simulink model "TrailerSoftware"  (R2019b)
settings: Solver=FixedStepDiscrete  StartTime=0.0  StopTime=inf  FixedStep=update  RelTol=1e-3  EnableMultiTasking=on
values from neighbouring files (symbols this model uses):
  countmax1 = 2500    [ProductionMfile.m]
  countmax2 = 2500    [ProductionMfile.m]
  HeaterIntGain = .0008    (= 0.0008)    [ProductionMfile.m]
  HeatGain = 10    [ProductionMfile.m]
  Intll = 0    [ProductionMfile.m]
  MaxCondPressure = 350    [ProductionMfile.m]
  MinSP = 1    [ProductionMfile.m]
  PostGain100 = 0.0002    [ProductionMfile.m]
  PostGain150 = 0.0005    [ProductionMfile.m]
  PostGain200 = 0.0004    [ProductionMfile.m]
  PostGain300 = 0.0008    [ProductionMfile.m]
  PostInit150 = 12    [ProductionMfile.m]
  PostIntulC = 65    [ProductionMfile.m]
  PostPGain = 0    [ProductionMfile.m]
  PreGain100 = 0.0005    [ProductionMfile.m]
  PreGain150 = 0.0005    [ProductionMfile.m]
  PreGain200 = 0.0003    [ProductionMfile.m]
  PreGain300 = 0.0008    [ProductionMfile.m]
  PreInit150 = 30    [ProductionMfile.m]
  PreIntulC = 65    [ProductionMfile.m]
  PreIntulDH = 65    [ProductionMfile.m]
  PrePGain = 0    [ProductionMfile.m]
  SatPress = [10 20 30 40 50 60 70 80 90 100 110 120 130 140 150 160 170      180 190 200 210 220 230 240 250 260 270 280 290 300 310 320 330      340 350 360 370 380 390 400 410 420 430 440 450 460 470 480 490      500]    [ProductionMfile.m]
  SatTemp = [-29.497 -2.4046 15.401 29.047 40.267 49.88 58.338 65.922 72.819      79.159 85.037 90.526 95.68 100.55 105.16 109.54 113.73 117.73 121.57      125.26 128.82 132.25 135.56 138.77 141.88 144.89 147.82 150.67 153.44      156.15 158.78 161.35 163.85 166.3 168.7 171.04 173.33 175.58 177.77      179.93 182.04 184.11 186.14 188.14 190.09 192.01 193.9 195.75 197.58      199.37]    [ProductionMfile.m]
  SHGain = 2    [ProductionMfile.m]
  SizeCANMatrix = 80    [ProductionMfile.m]
  SizeCOBIDVector = 10    [ProductionMfile.m]
  update = 0.002    [ProductionMfile.m]
undefined symbols (not defined in the file or in its folder): DiscIntNeverNeededParam, PostDGain, PreDGain, Ratio100, Ratio150, Ratio200, Ratio300
libraries: simulink x60, c2837xDlib x35, xpcutilitieslib x24, c2802xlib x8, c280xlib x7, etargetslib x4, svdutilitieslib x2, c2000lib x1
(part 2 of 8)

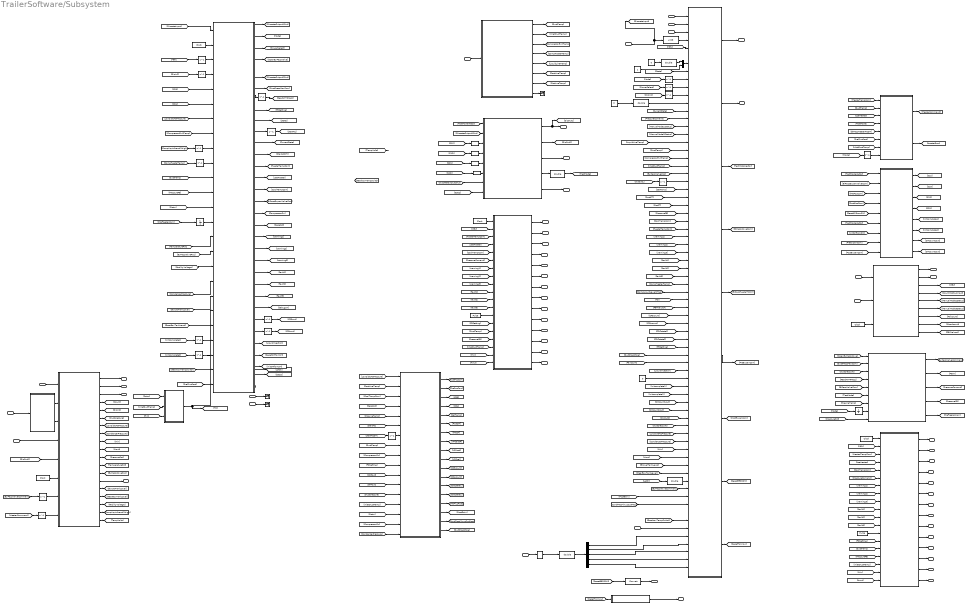
== system TrailerSoftware/Subsystem ==
  UDP Input Vector : Inport  OutDataTypeStr=uint8  PortDimensions=SizeUDPInput  SampleTime=update  LockScale=on
  A/D Vector : Inport  Port=2  PortDimensions=ADInputSize  SampleTime=update
  Discrete Input Word : Inport  Port=3  OutDataTypeStr=boolean  PortDimensions=DiscreteInputSize  SampleTime=update
  Modbus Input Vector : Inport  Port=4  OutDataTypeStr=uint8  PortDimensions=ModbusInputSize  SampleTime=update
  Modbus Input Ready : Inport  Port=5  OutDataTypeStr=uint8  PortDimensions=1  SampleTime=update
  UDP Input Ready : Inport  Port=6  OutDataTypeStr=boolean  PortDimensions=1  SampleTime=update
  CPUUtilizationsec : Inport  Port=7  OutDataTypeStr=double  PortDimensions=1  SampleTime=update
  EEPROM Input Vector : Inport  Port=8  OutDataTypeStr=single  PortDimensions=EEPROMSize  SampleTime=update
  New CAN Message : Inport  Port=9  OutDataTypeStr=uint8  SampleTime=update
  CAN Message Matrix : Inport  Port=10  OutDataTypeStr=uint8  PortDimensions=[1 SizeCANMatrix]  SampleTime=update
  CAN COBID Vector : Inport  Port=11  OutDataTypeStr=uint32  PortDimensions=[1 SizeCOBIDVector]  SampleTime=update
  RTD1 : Inport  Port=12  OutDataTypeStr=uint16  PortDimensions=1  SampleTime=update
  RTD2 : Inport  Port=13  OutDataTypeStr=uint16  PortDimensions=1  SampleTime=update
  WatchDogReset : Inport  Port=14  OutDataTypeStr=uint8  PortDimensions=1  SampleTime=update
  RomTestFailed : Inport  Port=15  OutDataTypeStr=uint8  PortDimensions=1  SampleTime=update
  CAN Process : MATLAB Function  TreatAsAtomicUnit=on
  Constant1 : Constant
  Constant2 : Constant  Value=0
  Constant4 : Constant  Value=0
  Constant9 : Constant  Value=0
  Data Type Conversion{1,8,10,12..13} (5 alike) : DataTypeConversion
  Data Type Conversion{2..3,6..7,9} (5 alike) : DataTypeConversion  OutDataTypeStr=double
  Data Type Conversion4 : DataTypeConversion  OutDataTypeStr=uint8
  Delay{,1..8,11..19} (18 alike) : Delay  DelayLength=1  InitialCondition=0
  Demux : Demux  Outputs=5
  Dew Point Temp : MATLAB Function  TreatAsAtomicUnit=on
  Digital Clock{,1..4} (5 alike) : DigitalClock  SampleTime=update
  Display : MATLAB Function  TreatAsAtomicUnit=on
  Display1 : MATLAB Function  TreatAsAtomicUnit=on
  Duct Pressure Control : Subsystem
  Heating : Subsystem
  MATLAB Function : MATLAB Function  TreatAsAtomicUnit=on
  Modbus Routine : MATLAB Function  TreatAsAtomicUnit=on
  Mux : Mux  Inputs=2
  Output Discrete : Subsystem
  Pulse Generator1 : DiscretePulseGenerator  Period=250  SampleTime=update
  Pulse Generator2 : DiscretePulseGenerator  Period=250  SampleTime=update
  Selector : Selector  InputPortWidth=32  IndexOptions=Index vector (dialog)  Indices=[28 29 30 31 32 ]  OutputSizes=1
  State Machine : MATLAB Function  TreatAsAtomicUnit=on
  Stepper Motor Reoutine : Subsystem
  Super Heat Control : Subsystem
  Temperature Vector : Subsystem
  Terminator3 : Terminator
  Terminator5 : Terminator
  Terminator6 : Terminator
  UDP Processing : Subsystem
  Unit Delay1 : UnitDelay  SampleTime=-1  HasFrameUpgradeWarning=on
  Unit Delay2 : UnitDelay  SampleTime=-1  HasFrameUpgradeWarning=on
  Unpack Data : Subsystem
  UDP Output Vector : Outport  OutDataTypeStr=uint8  PortDimensions=SizeUDPOutput  VectorParamsAs1DForOutWhenUnconnected=off  LockScale=on
  "Discrete Output Vector " : Outport  Port=2  OutDataTypeStr=uint8  PortDimensions=DiscreteOutputSize  SampleTime=update  VectorParamsAs1DForOutWhenUnconnected=off
  Modbus Output Vector : Outport  Port=3  OutDataTypeStr=uint8  PortDimensions=SizeModbusOutput  VectorParamsAs1DForOutWhenUnconnected=off  LockScale=on
  "HC Discrete Output Vector " : Outport  Port=4  OutDataTypeStr=uint8  PortDimensions=HCDiscreteOutputSize  SampleTime=update  VectorParamsAs1DForOutWhenUnconnected=off  LockScale=on
  Modbus Output Ready : Outport  Port=5  OutDataTypeStr=uint8  PortDimensions=1  SampleTime=update  VectorParamsAs1DForOutWhenUnconnected=off  LockScale=on
  UDP Output Ready : Outport  Port=6  OutDataTypeStr=uint8  SampleTime=update  VectorParamsAs1DForOutWhenUnconnected=off  LockScale=on
  Display Row 1 Char Array : Outport  Port=7  OutDataTypeStr=uint8  PortDimensions=SizeDisplayRow  SampleTime=update  VectorParamsAs1DForOutWhenUnconnected=off  LockScale=on
  Display Row 2 Char Array : Outport  Port=8  OutDataTypeStr=uint8  PortDimensions=SizeDisplayRow  SampleTime=update  VectorParamsAs1DForOutWhenUnconnected=off  LockScale=on
  Start Row 1 : Outport  Port=9  OutDataTypeStr=uint8  SampleTime=update  VectorParamsAs1DForOutWhenUnconnected=off  LockScale=on
  Start Row 2 : Outport  Port=10  OutDataTypeStr=uint8  SampleTime=update  VectorParamsAs1DForOutWhenUnconnected=off  LockScale=on
  Num Char Row 1 : Outport  Port=11  OutDataTypeStr=uint8  SampleTime=update  VectorParamsAs1DForOutWhenUnconnected=off  LockScale=on
  Num Char Row 2 : Outport  Port=12  OutDataTypeStr=uint8  SampleTime=update  VectorParamsAs1DForOutWhenUnconnected=off  LockScale=on
  Clear Display : Outport  Port=13  OutDataTypeStr=uint8  SampleTime=update  VectorParamsAs1DForOutWhenUnconnected=off  LockScale=on
  Display Data Available : Outport  Port=14  OutDataTypeStr=uint8  SampleTime=update  VectorParamsAs1DForOutWhenUnconnected=off  LockScale=on
  EEPROM Output Vector : Outport  Port=15  OutDataTypeStr=single  PortDimensions=EEPROMSize  SampleTime=update  VectorParamsAs1DForOutWhenUnconnected=off
  EEPROM Output Flag : Outport  Port=16  OutDataTypeStr=boolean  SampleTime=update  VectorParamsAs1DForOutWhenUnconnected=off
  Send CAN Message : Outport  Port=17  OutDataTypeStr=uint8  SampleTime=update  VectorParamsAs1DForOutWhenUnconnected=off
  CAN Data : Outport  Port=18  OutDataTypeStr=uint8  PortDimensions=SizeCANDataOut  SampleTime=update  VectorParamsAs1DForOutWhenUnconnected=off
  COBID : Outport  Port=19  OutDataTypeStr=uint32  SampleTime=update  VectorParamsAs1DForOutWhenUnconnected=off
  Number of bytes : Outport  Port=20  OutDataTypeStr=uint8  SampleTime=update  VectorParamsAs1DForOutWhenUnconnected=off
  Num Char Row 3 : Outport  Port=21  OutDataTypeStr=uint8  SampleTime=update  VectorParamsAs1DForOutWhenUnconnected=off  LockScale=on
  Num Char Row 4 : Outport  Port=22  OutDataTypeStr=uint8  SampleTime=update  VectorParamsAs1DForOutWhenUnconnected=off  LockScale=on
  Start Row 3 : Outport  Port=23  OutDataTypeStr=uint8  SampleTime=update  VectorParamsAs1DForOutWhenUnconnected=off  LockScale=on
  Start Row 4 : Outport  Port=24  OutDataTypeStr=uint8  SampleTime=update  VectorParamsAs1DForOutWhenUnconnected=off  LockScale=on
  Display Row 3 Char Array : Outport  Port=25  OutDataTypeStr=uint8  PortDimensions=SizeDisplayRow  SampleTime=update  VectorParamsAs1DForOutWhenUnconnected=off  LockScale=on
  Display Row 4 Char Array : Outport  Port=26  OutDataTypeStr=uint8  PortDimensions=SizeDisplayRow  SampleTime=update  VectorParamsAs1DForOutWhenUnconnected=off  LockScale=on
  Low Volt Discrete Output : Outport  Port=27  OutDataTypeStr=uint8  PortDimensions=SizeLowVoltDiscreteOutput  SampleTime=update  VectorParamsAs1DForOutWhenUnconnected=off
  Display Row 1 Char Array1 : Outport  Port=28  OutDataTypeStr=uint8  PortDimensions=SizeDisplayRow  SampleTime=update  VectorParamsAs1DForOutWhenUnconnected=off  LockScale=on
  Display Row 2 Char Array1 : Outport  Port=29  OutDataTypeStr=uint8  PortDimensions=SizeDisplayRow  SampleTime=update  VectorParamsAs1DForOutWhenUnconnected=off  LockScale=on
  Start Row 5 : Outport  Port=30  OutDataTypeStr=uint8  SampleTime=update  VectorParamsAs1DForOutWhenUnconnected=off  LockScale=on
  Start Row 6 : Outport  Port=31  OutDataTypeStr=uint8  SampleTime=update  VectorParamsAs1DForOutWhenUnconnected=off  LockScale=on
  Num Char Row 5 : Outport  Port=32  OutDataTypeStr=uint8  SampleTime=update  VectorParamsAs1DForOutWhenUnconnected=off  LockScale=on
  Num Char Row 6 : Outport  Port=33  OutDataTypeStr=uint8  SampleTime=update  VectorParamsAs1DForOutWhenUnconnected=off  LockScale=on
  Clear Display1 : Outport  Port=34  OutDataTypeStr=uint8  SampleTime=update  VectorParamsAs1DForOutWhenUnconnected=off  LockScale=on
  Display Data Available1 : Outport  Port=35  OutDataTypeStr=uint8  SampleTime=update  VectorParamsAs1DForOutWhenUnconnected=off  LockScale=on
  Num Char Row 7 : Outport  Port=36  OutDataTypeStr=uint8  SampleTime=update  VectorParamsAs1DForOutWhenUnconnected=off  LockScale=on
  Num Char Row 8 : Outport  Port=37  OutDataTypeStr=uint8  SampleTime=update  VectorParamsAs1DForOutWhenUnconnected=off  LockScale=on
  Start Row 7 : Outport  Port=38  OutDataTypeStr=uint8  SampleTime=update  VectorParamsAs1DForOutWhenUnconnected=off  LockScale=on
  Start Row 8 : Outport  Port=39  OutDataTypeStr=uint8  SampleTime=update  VectorParamsAs1DForOutWhenUnconnected=off  LockScale=on
  Display Row 3 Char Array1 : Outport  Port=40  OutDataTypeStr=uint8  PortDimensions=SizeDisplayRow  SampleTime=update  VectorParamsAs1DForOutWhenUnconnected=off  LockScale=on
  Display Row 4 Char Array1 : Outport  Port=41  OutDataTypeStr=uint8  PortDimensions=SizeDisplayRow  SampleTime=update  VectorParamsAs1DForOutWhenUnconnected=off  LockScale=on
  wires:
  [GearboxTempSwitch] -> UDP Processing/65(GearBoxTemp)
  Modbus Routine/5(ManualMode2StatusOut) -> [ManualMode2Status]
  Output Discrete/1("Discrete Output Vector 1 ") -> [DisOut1], "Discrete Output Vector "/1
  Heating/2(Heater Error) -> [HeaterError]
  Temperature Vector/1(Outlet Duct Temperature) -> [DuctTemp]
  [CompHeaterTemp] -> UDP Processing/35(HeaterTemp)  "36"
  [ResetToKnow] -> MATLAB Function/1(settoknown)
  Super Heat Control/14(CDCstate2) -> [CDCstate2]
  Output Discrete/5(Low Volt Discrete Output) -> Low Volt Discrete Output/1
  ? -> [GearboxTempSwitch]
  UDP Processing/8(Reset EEPROM) -> [ResetEEPROM]
  Super Heat Control/16(PostGain) -> [PostGain]
  Delay19/1 -> Heating/8(Tmode1)
  [PressureFB] -> State Machine/12(PressureFB)
  UDP Processing/9(Reset to Known) -> [ResetToKnow]
  State Machine/30(InitSM) -> [InitSMfromSM]
  [CompressorExitTemp] -> State Machine/8(CompExitTemp)
  [CondenserPressure] -> UDP Processing/55(Condensor Pressure)  "56"
  Temperature Vector/3(Compressor Exit Temperature) -> [CompressorExitTemp]
  [Initcomplete1] -> UDP Processing/48(Init1complete)  "49"
  RTD1/1 -> Terminator5/1
  Delay18/1 -> State Machine/22(Initcomplete2)
  MATLAB Function/1(y) -> EEPROM Output Vector/1
  [BlowerTankLevel] -> UDP Processing/58(BlowerTankLevel)  "59"
  [FRSetting] -> Super Heat Control/10(FR)
  Delay12/1 -> [CR4out]
  [Mode] -> Delay19/1
  [LowSideACPressure] -> State Machine/7(SuctionPressure)
  [CoolTempCom] -> Display/5(CoolTempCom)
  [Patm] -> State Machine/13(Patm)
  UDP Processing/2(UDP Output Ready) -> UDP Output Ready/1
  [PrePlusPost] -> State Machine/25(PrePlusPost)
  State Machine/31(Latch) -> [Latch]
  Data Type Conversion12/1 -> Output Discrete/5(Post Step)
  [TestMode] -> Duct Pressure Control/6(TestMode)
  Data Type Conversion9/1 -> Demux/1
  [PressureFB] -> UDP Processing/26(Pressure FB)  "26"
  [TempVolts] -> ?
  Duct Pressure Control/5(PreFreezeWarn) -> [PreFreezeWarn]
  Duct Pressure Control/2(Ambient Pressure) -> [Patm]
  Data Type Conversion6/1 -> UDP Processing/12(Debug)
  State Machine/21(warning3) -> [warning3]
  [DuctPressPsig] -> UDP Processing/44(GoodCount)  "45"
  [InletDuctTemp] -> Heating/7(Tamb)
  State Machine/7(ReadATMPress) -> Delay2/1
  CAN Process/7(LowSideACPressureOut) -> [LowSideACPressure]
  [CR4] -> State Machine/6(CR4)
  CAN Process/2(CANData) -> CAN Data/1
  Temperature Vector/7(Pre Line Temperature) -> [PreLineTemp]
  [InletDuctTemp] -> Dew Point Temp/2(Tinlet)
  [PressurePot] -> Duct Pressure Control/9(Pressure Pot)
  [DuctTemp] -> Super Heat Control/8(DuctTemp)
  RTD2/1 -> Terminator6/1
  [Hin] -> Dew Point Temp/3(Rh)
  Constant2/1 -> Data Type Conversion6/1
  [PostGain] -> UDP Processing/62(Heater Error)
  [CR4out] -> Super Heat Control/12(CR4out)
  [CompressorOn] -> Super Heat Control/16(CoolingMode)
  Data Type Conversion7/1 -> UDP Processing/60(Latch)
  State Machine/10(StartAC) -> Delay4/1
  Super Heat Control/13(CDCstate1) -> [CDCstate1]
  [Initcomplete1] -> Delay17/1
  [estop] -> Output Discrete/8(estop)
  [warning2] -> UDP Processing/30(warning2)  "30"
  [StartACDH] -> Delay8/1
  [PostST] -> UDP Processing/24(PostST)  "24"
  [warning3] -> UDP Processing/31(warning3)  "31"
  State Machine/24(fault3) -> [fault3]
  [DisOut1] -> Delay11/1
  [DisOut2] -> UDP Processing/52(DisOut2)  "53"
  CAN Process/14(SendCANMessage) -> Send CAN Message/1
  Modbus Routine/3(ModbusVector) -> [MBV]
  [CR3] -> State Machine/5(CR3)
  State Machine/19(warning1) -> [warning1]
  State Machine/1(OutputDiscretes1Out) -> [DiscreteOutput1Out]
  [Hin] -> Display/18(Hin)
  CAN Process/17(FacilityVoltageOut) -> [FacilityVoltage]
  Data Type Conversion3/1 -> [TestMode]
  [ByPassValvePos] -> State Machine/16(ByPassValvePos)
  [GearBoxTankLevel] -> State Machine/20(GearBoxLevel)
  [warning1] -> UDP Processing/29(warning1)  "29"
  State Machine/14(UseHeater) -> [UseHeater]
  Display/4(DisRow4) -> Display Row 4 Char Array/1
  [TD] -> UDP Processing/37(TD)  "38"
  CAN Process/13(ByPassValvePosOut) -> [ByPassValvePos]
  [CR4count] -> UDP Processing/40(CR4count)  "41"
  [PressureFB] -> Display/16(DuctPress)
  CAN Process/1(COBID) -> COBID/1
  CAN Process/16(GearBoxTankLevelSensorOut) -> [GearBoxTankLevel]
  Digital Clock3/1 -> CAN Process/6(time)
  [CondenserPressure] -> State Machine/18(CondenserPressure)
  [BiPassValveCom] -> Duct Pressure Control/5(BiPassPosCom)
  [CDCstate1] -> UDP Processing/41(CDCstate1)  "42"
  [DuctTemp] -> Display/15(DuctTemp)
  Duct Pressure Control/1("ByPass Valve Command % ") -> [ByPassValveCommand]
  State Machine/5(OutputDiscretes2Out) -> [DiscreteOutput2Out]
  Selector/1 -> Data Type Conversion9/1
  Temperature Vector/8(Spare Temperature) -> Terminator3/1
  Display/13(ClearDisplay) -> Clear Display/1
  CAN Process/11(PressurePotOut) -> [PressurePot]
  Delay3/1 -> UDP Processing/11(Discrete Input Vector 2)  "11"
  [ByPassValveCommand] -> Delay16/1
  Data Type Conversion13/1 -> Output Discrete/6(PostDir)
  UDP Input Vector/1 -> UDP Processing/1(UDP Input Vector)  "1"
  Delay8/1 -> Super Heat Control/7(StartACDH)
  Delay11/1 -> UDP Processing/22(DisOut1)  "22"
  EEPROM Input Vector/1 -> Selector/1
  Data Type Conversion10/1 -> Output Discrete/3(Pre Step)
  [HeaterTempCom] -> Display/3(HeaterTempCom)
  [HeaterCommand] -> Delay7/1
  Output Discrete/2(Discrete Output Vector 2) -> [DisOut2]
  Modbus Routine/8(Goodcountout) -> [Goodcount]
  State Machine/29(ResetSM) -> [ResetSMfromSM]
  [GearboxTempSwitch] -> State Machine/24(GearboxTempSwitch)
  [SMcount1out] -> UDP Processing/50(SMcount1)  "51"
  [UseHeater] -> Heating/3(UseHeater)
  Unit Delay1/1 -> State Machine/14(PreFreezeWarn)
  [CoolTempCom] -> Super Heat Control/3(TempCom)
  [PreFreezeWarn] -> Unit Delay1/1
  Super Heat Control/2(Pre Pos Com) -> [PrePosCom]
  State Machine/26(CR3out) -> Delay13/1
  [CondenserPressure] -> Super Heat Control/17(Condenser Pressure1)
  CAN Message Matrix/1 -> Unpack Data/1(In1)
  Display/3(DisRow3) -> Display Row 3 Char Array/1
  Demux/5 -> UDP Processing/71(EEPROM 32)
  [InletDuctTemp] -> UDP Processing/20(InletDuctTemp)  "20"
  Display/6(StartRow2) -> Start Row 2/1
  State Machine/6(MaxPressureout) -> [DuctPressMaxCom]
  Display/8(StartRow4) -> Start Row 4/1
  [FRSetting] -> Display/14(FlowRate)
  Display/7(StartRow3) -> Start Row 3/1
  [HeaterTempCom] -> UDP Processing/28(Heater Temp Command)  "28"
  [FacilityVoltage] -> State Machine/17(FacilityVoltage)
  Super Heat Control/12(CR4count) -> [CR4count]
  Delay16/1 -> CAN Process/7(BiPassValveCom)
  Demux/2 -> UDP Processing/68(EEPROM 29)
  Super Heat Control/10(VPPreI) -> [VPPreI]
  Data Type Conversion2/1 -> Mux/1
  Display/12(NumCharRow4) -> Num Char Row 4/1
  Display/11(NumCharRow3) -> Num Char Row 3/1
  WatchDogReset/1 -> UDP Processing/66(WatchDogReset)
  [CompHeaterTemp] -> Delay14/1
  Modbus Routine/9(FaultBitMapValueAOut) -> [FBMValueA]
  Temperature Vector/2(Inlet Duct Temperature) -> [InletDuctTemp]
  [CoolTempCom] -> UDP Processing/27(Cool Temp Command)  "27"
  [DuctTemp] -> State Machine/11(DuctTemp)
  CAN Process/3(NumBytes) -> Number of bytes/1
  [LiquidInjection] -> UDP Processing/46(LiquidInjection)  "47"
  State Machine/25(debugout) -> [debugsm]
  [DiscreteOutput1Out] -> Output Discrete/2(Discrete Output from State machine 1)
  Super Heat Control/17(CondPresMinusSucPres) -> [CondPresMinusSucPres]
  Pulse Generator2/1 -> Display/13(Pulse)
  [Mode] -> Unit Delay2/1
  Delay14/1 -> State Machine/10(CompHeaterTemp)
  [Failcount] -> UDP Processing/45(FailCount)  "46"
  [PreLineTemp] -> Duct Pressure Control/7(PreSuctionTemp)
  [Hin] -> UDP Processing/56(Hin)  "57"
  [CompLiquidLevel2High] -> Delay15/1
  CAN Process/18(CompressorLevelOut) -> [CompLiquidLevel2High]
  State Machine/23(fault2) -> [fault2]
  [CR3out] -> Super Heat Control/11(CR3out)
  Delay13/1 -> [CR3out]
  State Machine/22(fault1) -> [fault1]
  [MBV] -> Display/2(MBV)
  [Ductpressure] -> Super Heat Control/13(Ductpresspsia)
  [Patm] -> Super Heat Control/15(Patm)
  [LowSideACPressure] -> UDP Processing/54(Suction Pressure)  "55"
  Delay15/1 -> State Machine/9(CompLiquidLevel2High)
  [ReadATMPress] -> Duct Pressure Control/4(Read ATM Pressure)
  [fault3] -> UDP Processing/34(fault3)  "34"
  Delay2/1 -> [ReadATMPress]
  CAN Process/10(HumiditySensorOutOut) -> [Hout]
  [Latch] -> Data Type Conversion7/1  "61"
  [CompressorOn] -> Super Heat Control/9(CompressorOn)
  State Machine/27(CR4out) -> Delay12/1
  A/D Vector/1 -> Temperature Vector/1(In1)
  [fault2] -> Display/11(fault2)
  [UseHeater] -> Display/4(UseHeater)
  Display/1(DisRow1) -> Display Row 1 Char Array/1
  State Machine/13(HeaterTempCom) -> [HeaterTempCom]
  CAN Process/19(voltsout) -> [TempVolts]
  Unit Delay2/1 -> Duct Pressure Control/8(Mode)
  [warning3] -> Display/9(warning3)
  [Hout] -> UDP Processing/57(Hout)  "58"
  State Machine/9(stateout) -> [State]
  CAN Process/8(ACCondenserPressureOut) -> [CondenserPressure]
  Display/10(NumCharRow2) -> Num Char Row 2/1
  [ResetAC] -> Super Heat Control/4(Reset)
  [warning1] -> Display/7(warning1)
  [CR3count] -> UDP Processing/39(CR3count)  "40"
  [fault2] -> UDP Processing/33(fault2)  "33"
  [fault1] -> UDP Processing/32(fault1)  "32"
  [Ductpressure] -> UDP Processing/53(Duct Pressure)  "54"
  [fault3] -> Display/12(fault3)
  Output Discrete/4(TestMode) -> Data Type Conversion3/1
  State Machine/17(CompressorOnOut) -> [CompressorOn]
  Delay17/1 -> State Machine/21(Initcomplete1)
  Display/2(DisRow2) -> Display Row 2 Char Array/1
  Modbus Input Ready/1 -> Modbus Routine/1(ModbusInputReady)
  [PreLineTemp] -> Super Heat Control/5(Pre Suction Temp)
  [Initcomplete2] -> UDP Processing/49(Init2complete)  "50"
  [BlowerTankLevel] -> State Machine/19(BlowerLevel)
  Super Heat Control/11(CR3count) -> [CR3count]
  [Ductpressure] -> Duct Pressure Control/3(Duct Pressure)
  Temperature Vector/4(Compressor Heater Temperature) -> [CompHeaterTemp]
  [ByPassValveCommand] -> UDP Processing/61(ByPassValvePosCmd)
  [DisOut2] -> CAN Process/5(DisOut2)
  [Patm] -> Dew Point Temp/1(Patm)
  [DisIn2] -> Delay3/1
  Data Type Conversion1/1 -> EEPROM Output Flag/1
  Digital Clock/1 -> Modbus Routine/3(time)
  [Initcomplete2] -> Delay18/1
  [DuctTemp] -> Heating/2(Duct Temp)
  Modbus Routine/7(Failcountout) -> [Failcount]
  Demux/1 -> UDP Processing/67(EEPROM 28)
  Heating/1(Heater Command) -> [HeaterCommand]
  [CompLiquidLevel2High] -> UDP Processing/36(Liquid Level)  "37"
  Constant4/1 -> Data Type Conversion2/1
  [CurrentState] -> UDP Processing/13(Current State)  "13"
  Super Heat Control/1(Post Pos Com) -> [PostPosCom]
  [BiPassHeaterTCOM] -> Heating/5(BiPassHeatCom)
  [ResetEEPROM] -> Data Type Conversion1/1
  [TestMode] -> Heating/4(Test Mode)
  [PressureComand] -> Display/6(PressCommand)
  [TemperaturePot] -> State Machine/15(TempPot)
  [State] -> UDP Processing/8(State)  "9"
  Delay4/1 -> [StartAC]
  UDP Processing/3(Test Mode Vector 1) -> [TestModeVector]
  CAN Process/12(TemperaturePotOut) -> [TemperaturePot]
  UDP Processing/5(BiPass Heater Temp Command) -> [BiPassHeaterTCOM]
  CAN Process/6(DuctpressureOut) -> [Ductpressure]
  CAN Process/5(DisIn2Out) -> [DisIn2]
  State Machine/16(BiPassExpanValveCom) -> [BiPassExpanValveCom]
  [ManualMode3Status] -> UDP Processing/16(MM3Status)  "16"
  Duct Pressure Control/4(Pressure Feedback) -> [PressureFB]
  Demux/4 -> UDP Processing/70(EEPROM 31)
  [StartAC] -> Super Heat Control/6(StartAC)
  [warning2] -> Display/8(warning2)
  CAN Process/9(HumiditySensorInOut) -> [Hin]
  UDP Processing/4(BiPass Valve Pos Command) -> [BiPassValveCom]
  Modbus Routine/2(ModbusOutVector) -> Modbus Output Vector/1
  [LowSideACPressure] -> Super Heat Control/1("Suction Pressure, psia")
  Delay6/1 -> State Machine/3(MBV)
  State Machine/12(StartACDH) -> [StartACDH]
  State Machine/8(FRSettingOut) -> [FRSetting]
  Delay5/1 -> State Machine/4(DiscreteInput2)
  [InletDuctTemp] -> Display/17(DuctTempIn)
  State Machine/11(CurrentStateOut) -> [CurrentState]
  [SMcount2out] -> UDP Processing/51(SMcount2)  "52"
  [fault1] -> Display/10(fault1)
  [DisIn2] -> Delay5/1
  Super Heat Control/9(VPPostI) -> [VPPostI]
  Digital Clock1/1 -> Display/1(time)
  Super Heat Control/6(Post Superheat Temp) -> [PostST]
  Super Heat Control/8(VPdeltaP) -> [VPdeltaP]
  Demux/3 -> UDP Processing/69(EEPROM 30)
  [Mode] -> Delay/1
  Display/9(NumCharRow1) -> Num Char Row 1/1
  Discrete Input Word/1 -> [DiscreteInput], Data Type Conversion4/1
  Super Heat Control/5(Satutation Temp) -> [SatTemp]
  [FRSetting] -> UDP Processing/43(FRSetting)  "44"
  Super Heat Control/4(CR4) -> [CR4]
  Super Heat Control/15(PrePlusPost) -> [PrePlusPost]
  [ManualMode2Status] -> UDP Processing/15(MM2Status)  "15"
  Modbus Routine/4(countoutputout) -> [CountModbusInput]
  State Machine/18(ResetAC) -> [ResetAC]
  [PrePlusPost] -> Heating/6(PrePlusPost)
  [PostLineTemp] -> Super Heat Control/2(Post Suction Temp)
  Dew Point Temp/1(td) -> [TD], State Machine/23(td)
  [CompressorExitTemp] -> UDP Processing/19(CompressorExitTemp)  "19"
  UDP Processing/6("Pre Expansion Valve, %") -> [PreExpanCom]
  [FBMValueA] -> UDP Processing/38(FaultMapA)  "39"
  State Machine/32(estopout) -> [estop]
  [PressureComand] -> UDP Processing/14(Pressure Command)  "14"
  [ByPassValvePos] -> UDP Processing/21(ByPassValvePos)  "21"
  [PreST] -> UDP Processing/25(PreST)  "25"
  CAN Process/4(CountOut) -> [Count]
  Delay7/1 -> CAN Process/8(HeaterCom)
  State Machine/15(CoolTempCom) -> [CoolTempCom]
  Unpack Data/2(Lower) -> CAN Process/3(CANDataLower)
  Display/14(DisplayDataAvail) -> Display Data Available/1
  Data Type Conversion4/1 -> UDP Processing/4(Discrete Input Vector 1)  "4"
  Modbus Routine/6(ManualMode3StatusOut) -> [ManualMode3Status]
  [TestModeVector] -> Output Discrete/1(Test Mode Vector 1)
  [SatTemp] -> UDP Processing/23(SatTemp)  "23"
  [DuctTemp] -> UDP Processing/18(Duct Temperature)  "18"
  [Hout] -> Display/19(Hout)
  [LiquidLineTemp] -> UDP Processing/17(Condenser Temp)  "17"
  [OpenByPassValve] -> Duct Pressure Control/1(Open ByPassValve)
  New CAN Message/1 -> CAN Process/1(NewCANMessage)
  [MBV] -> Delay6/1
  Constant9/1 -> UDP Processing/47(LowOilFlag)  "48"
  Mux/1 -> UDP Processing/7(Memory)  "7-8"
  Constant1/1 -> Mux/2
  Delay1/1 -> UDP Processing/10(Power Select)  "10"
  Delay/1 -> UDP Processing/9(Mode)  "9"
  Duct Pressure Control/3(Pressure Command,psig) -> [PressureComand]
  Super Heat Control/7(Pre Superheat Temp) -> [PreST]
  State Machine/3(powerselectout) -> [PowerSelect]
  Modbus Input Vector/1 -> Modbus Routine/2(ModbusInputVector)
  Super Heat Control/3(CR3) -> [CR3]
  [DiscreteOutput2Out] -> Output Discrete/7(Discrete Output from State machine 2)
  [PowerSelect] -> Delay1/1
  State Machine/2(modeout) -> [Mode]
  CAN Process/15(BlowerTankLevelSensorOut) -> [BlowerTankLevel]
  UDP Input Ready/1 -> UDP Processing/3(UDP Input Ready)  "3"
  Data Type Conversion8/1 -> Output Discrete/4(Pre Dir)
  UDP Processing/1(UDP Output) -> UDP Output Vector/1
  State Machine/28(LiquidInjectionOnOut) -> [LiquidInjection]
  [MBV] -> UDP Processing/5(MBV)  "5"
  [InletDuctTemp] -> Super Heat Control/14(Tin)
  State Machine/4(OpenByPassValve) -> [OpenByPassValve]
  [DuctPressMaxCom] -> Duct Pressure Control/2("Duct Pressure Max Com, psig")
  [DiscreteInput] -> State Machine/1(DiscreteInput1)
  Temperature Vector/6(Post Line Temperature) -> [PostLineTemp]
  Modbus Routine/1(ModbusOutReady) -> Modbus Output Ready/1
  Digital Clock2/1 -> State Machine/2(time)
  State Machine/20(warning2) -> [warning2]
  CPUUtilizationsec/1 -> UDP Processing/2(CPU Utilization sec)  "2"
  Display/5(StartRow1) -> Start Row 1/1
  Unpack Data/1(Upper) -> CAN Process/2(CANDataUpper)
  [HeaterTempCom] -> Heating/1(Heater Command Temp)
  Temperature Vector/5(Liquid Line Temperature) -> [LiquidLineTemp]
  Output Discrete/3("HC Discrete Output Vector ") -> "HC Discrete Output Vector "/1
  [CDCstate2] -> UDP Processing/42(CDCstate2)  "43"
  [GearBoxTankLevel] -> UDP Processing/59(GearBoxLevel)  "60"
  UDP Processing/7("Post Expansion Valve, %") -> [PostExpanCom]
  CAN COBID Vector/1 -> CAN Process/4(CANCOBIDVec)
  [CondPresMinusSucPres] -> UDP Processing/63(Debug4)
  [TestModeVector] -> Stepper Motor Reoutine/1(Test Mode Vector)
  [BiPassExpanValveCom] -> Stepper Motor Reoutine/2(BiPass Expan Valve Com)
  [PrePosCom] -> Stepper Motor Reoutine/3(Pre-Pos Com)
  [PostPosCom] -> Stepper Motor Reoutine/4(Post Pos Com)
  [ResetSMfromSM] -> Stepper Motor Reoutine/5(Reset SM from SM)
  [TestModeVector] -> Stepper Motor Reoutine/6(Reset SM from SM)
  [InitSMfromSM] -> Stepper Motor Reoutine/7(Init SM from SM)
  Stepper Motor Reoutine/1(S1S) -> [S1S]
  [S1D] -> Data Type Conversion8/1
  Stepper Motor Reoutine/3(S2S) -> [S2S]
  [S2D] -> Data Type Conversion13/1
  Stepper Motor Reoutine/5(Init 1 Complete) -> [Initcomplete1]
  Stepper Motor Reoutine/6(Init 2 Complete) -> [Initcomplete2]
  Stepper Motor Reoutine/7(CNT 1 Out) -> [SMcount1out]
  Stepper Motor Reoutine/8(CNT 2 Out) -> [SMcount2out]
  [PreExpanCom] -> Stepper Motor Reoutine/8(Pre SM Com)
  [PostExpanCom] -> Stepper Motor Reoutine/9(PostSM Com)
  Stepper Motor Reoutine/4(S2D) -> [S2D]
  [S2S] -> Data Type Conversion12/1
  Stepper Motor Reoutine/2(S1D) -> [S1D]
  [S1S] -> Data Type Conversion10/1
  [PressureFB] -> Display1/16(DuctPress)
  [DuctTemp] -> Display1/15(DuctTemp)
  Display1/14(DisplayDataAvail) -> Display Data Available1/1
  [Hin] -> Display1/18(Hin)
  [HeaterTempCom] -> Display1/3(HeaterTempCom)
  [warning2] -> Display1/8(warning2)
  Display1/5(StartRow1) -> Start Row 5/1
  Display1/13(ClearDisplay) -> Clear Display1/1
  Display1/10(NumCharRow2) -> Num Char Row 6/1
  [Hout] -> Display1/19(Hout)
  [InletDuctTemp] -> Display1/17(DuctTempIn)
  [fault1] -> Display1/10(fault1)
  Display1/9(NumCharRow1) -> Num Char Row 5/1
  [fault3] -> Display1/12(fault3)
  Display1/2(DisRow2) -> Display Row 2 Char Array1/1
  [warning1] -> Display1/7(warning1)
  Display1/1(DisRow1) -> Display Row 1 Char Array1/1
  [PressureComand] -> Display1/6(PressCommand)
  Display1/3(DisRow3) -> Display Row 3 Char Array1/1
  [fault2] -> Display1/11(fault2)
  [MBV] -> Display1/2(MBV)
  Display1/12(NumCharRow4) -> Num Char Row 8/1
  Display1/7(StartRow3) -> Start Row 7/1
  Display1/8(StartRow4) -> Start Row 8/1
  Display1/6(StartRow2) -> Start Row 6/1
  [CoolTempCom] -> Display1/5(CoolTempCom)
  Display1/11(NumCharRow3) -> Num Char Row 7/1
  [warning3] -> Display1/9(warning3)
  [FRSetting] -> Display1/14(FlowRate)
  Pulse Generator1/1 -> Display1/13(Pulse)
  Digital Clock4/1 -> Display1/1(time)
  Display1/4(DisRow4) -> Display Row 4 Char Array1/1
  [UseHeater] -> Display1/4(UseHeater)
  Super Heat Control/18("Duct Pressure, PSIG") -> [DuctPressPsig]

== system TrailerSoftware/UIRec ==
  SCI_Rx_INT : TriggerPort  TriggerType=function-call  VariantControl=Variant
  Byte Pack : etargetslib/Byte Pack  datatypes={'uint32'}  byteAlign=1
      settings: SourceProductName=MATLAB Coder
  Byte Reversal : etargetslib/Byte Reversal  numInp=1
      settings: SourceProductName=MATLAB Coder  SourceProductBaseCode=ME
  Byte Unpack1 : etargetslib/Byte Unpack  dimensions={[5]}  datatypes={'single'}  byteAlign=1
      settings: SourceProductName=MATLAB Coder
  Logical Operator : Logic  AllPortsSameDT=off  OutDataTypeStr=boolean
  SCI Receive : c280xlib/SCI Receive  sciModule=B  dataHead='S'  dataTail='E'  dataType=uint32  dataDim=5  initValue=0  errOption=Output the last received value  errValue=0  sampleTime=-1  outputStatus=on  postInterrupt=on  numFifo=2
      settings: SourceProductName=Embedded Coder Support Package for Texas Instruments C2000 Processors  SourceProductBaseCode=TIC2000
  Selector1 : Selector  InputPortWidth=5  IndexOptions=Index vector (dialog)  Indices=[1 2 3 4]  OutputSizes=1
  Selector2 : Selector  InputPortWidth=5  IndexOptions=Index vector (dialog)  Indices=[1 2 3 4]  OutputSizes=1
  Selector3 : Selector  InputPortWidth=5  IndexOptions=Index vector (dialog)  Indices=[5]  OutputSizes=1
  Sum of Elements : Sum  Inputs=+
  Data From UI : Outport
  CheckSumOK : Outport  Port=2
  Out1 : Outport  Port=3
  wires:
  SCI Receive/2 -> Out1/1
  SCI Receive/1 -> Byte Reversal/1
  Byte Reversal/1 -> Selector1/1, Selector3/1, Byte Pack/1
  Byte Pack/1 -> Byte Unpack1/1
  Selector1/1 -> Sum of Elements/1
  Sum of Elements/1 -> Logical Operator/1
  Byte Unpack1/1 -> Selector2/1
  Selector2/1 -> Data From UI/1
  Selector3/1 -> Logical Operator/2
  Logical Operator/1 -> CheckSumOK/1

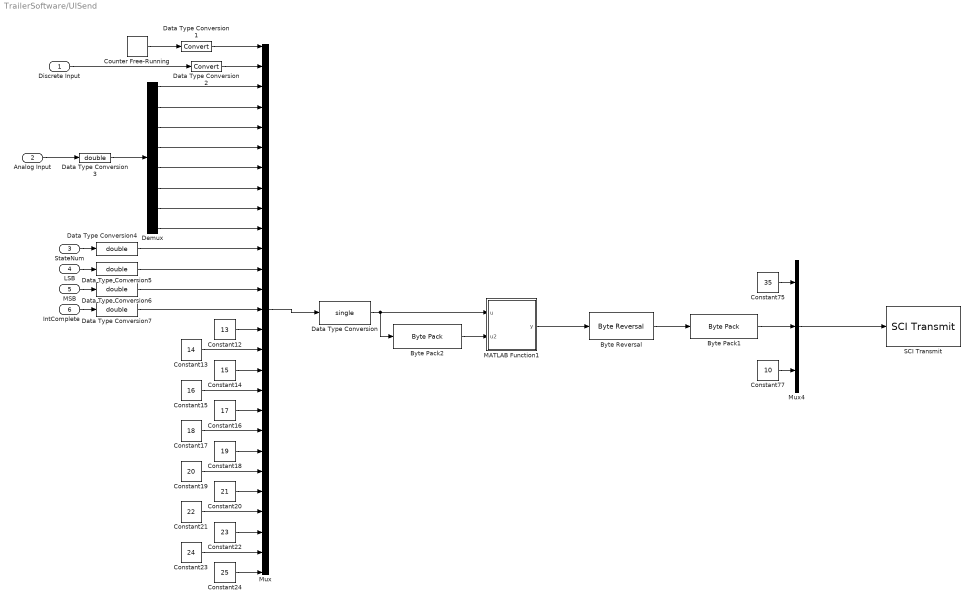
== system TrailerSoftware/UISend ==
  " Discrete Input" : Inport
  Analog Input : Inport  Port=2
  StateNum : Inport  Port=3
  LSB : Inport  Port=4
  MSB : Inport  Port=5
  IntComplete : Inport  Port=6
  Byte Pack1 : svdutilitieslib/Byte Pack  maskPackedDataType=uint8  datatypes={'single'}  byteAlign=1  blockPlatform=tic2000
      settings: SourceProductName=Embedded Coder Support Package for ARM Cortex-A Processors  SourceProductBaseCode=ECCORTEXA
  Byte Pack2 : svdutilitieslib/Byte Pack  maskPackedDataType=uint8  datatypes={'single'}  byteAlign=1  blockPlatform=tic2000
      settings: SourceProductName=Embedded Coder Support Package for ARM Cortex-A Processors  SourceProductBaseCode=ECCORTEXA
  Byte Reversal : etargetslib/Byte Reversal  numInp=1
      settings: SourceProductName=MATLAB Coder  SourceProductBaseCode=ME
  Constant12 : Constant  Value=13
  Constant13 : Constant  Value=14
  Constant14 : Constant  Value=15
  Constant15 : Constant  Value=16
  Constant16 : Constant  Value=17
  Constant17 : Constant  Value=18
  Constant18 : Constant  Value=19
  Constant19 : Constant  Value=20
  Constant20 : Constant  Value=21
  Constant21 : Constant  Value=22
  Constant22 : Constant  Value=23
  Constant23 : Constant  Value=24
  Constant24 : Constant  Value=25
  Constant75 : Constant  Value=35  OutDataTypeStr=uint8
  Constant77 : Constant  Value=10  OutDataTypeStr=uint8
  Counter Free-Running : simulink/Sources/Counter Free-Running  NumBits=16  tsamp=-1
  Data Type Conversion : DataTypeConversion  OutDataTypeStr=single
  Data Type Conversion1 : DataTypeConversion
  Data Type Conversion2 : DataTypeConversion
  Data Type Conversion{3..7} (5 alike) : DataTypeConversion  OutDataTypeStr=double
  Demux : Demux  Outputs=8
  MATLAB Function1 : MATLAB Function
  Mux : Mux  Inputs=27
  Mux4 : Mux  Inputs=3
  SCI Transmit : c280xlib/SCI Transmit  sciModule=B  dataHead=''  dataTail=''  postInterrupt=off  numFifo=16
      settings: SourceProductName=Embedded Coder Support Package for Texas Instruments C2000 Processors
  wires:
  Data Type Conversion1/1 -> Mux/1
  Demux/1 -> Mux/3
  Demux/3 -> Mux/5
  Demux/5 -> Mux/7
  Data Type Conversion5/1 -> Mux/12
  Data Type Conversion6/1 -> Mux/13
  Data Type Conversion7/1 -> Mux/14
  Constant12/1 -> Mux/15
  Constant13/1 -> Mux/16
  Constant14/1 -> Mux/17
  Constant15/1 -> Mux/18
  Constant16/1 -> Mux/19
  Constant17/1 -> Mux/20
  Constant18/1 -> Mux/21
  Constant19/1 -> Mux/22
  Constant20/1 -> Mux/23
  Constant21/1 -> Mux/24
  Constant22/1 -> Mux/25
  Constant23/1 -> Mux/26
  Constant24/1 -> Mux/27
  Data Type Conversion/1 -> Byte Pack2/1, MATLAB Function1/1(u)
  Byte Pack2/1 -> MATLAB Function1/2(u2)
  MATLAB Function1/1(y) -> Byte Reversal/1
  Byte Pack1/1 -> Mux4/2
  Constant75/1 -> Mux4/1
  Constant77/1 -> Mux4/3
  Byte Reversal/1 -> Byte Pack1/1
  Counter Free-Running/1 -> Data Type Conversion1/1
  " Discrete Input"/1 -> Data Type Conversion2/1
  Data Type Conversion2/1 -> Mux/2
  Demux/2 -> Mux/4
  Demux/4 -> Mux/6
  Demux/6 -> Mux/8
  Mux/1 -> Data Type Conversion/1
  Analog Input/1 -> Data Type Conversion3/1
  Data Type Conversion3/1 -> Demux/1
  StateNum/1 -> Data Type Conversion4/1
  Demux/7 -> Mux/9
  Demux/8 -> Mux/10
  Mux4/1 -> SCI Transmit/1
  Data Type Conversion4/1 -> Mux/11
  LSB/1 -> Data Type Conversion5/1
  MSB/1 -> Data Type Conversion6/1
  IntComplete/1 -> Data Type Conversion7/1

== system TrailerSoftware/SPI Interface/Chart/Address ==
  value : Inport  OutDataTypeStr=uint16  PortDimensions=1
  f : TriggerPort  TriggerType=function-call  VariantControl=(inherit)
      settings: CopyFcn=Stateflow.SLINSF.SimulinkMan.removeBlockPreDeleteFcn  PreDeleteFcn=Stateflow.SLINSF.SimulinkMan.unsafePredeleteFcn
  SPI Master Transfer : c280xlib/SPI Master Transfer  SPISelect=SPI_A  ClockPolarity=Rising_edge  ClockPhase=No_delay  SPIModule=uint32(0)  Mode=Master  BusSpeed=uint32(1000000)  FirstBitToTransfer=Most significant bit (MSB)  ClockMode=0  BlockFunction=Transfer  EnableRegisterAddress=off  RegisterAddress=0  OutputDataType=int8  OutputDataLength=1  DataBits=8  UseCustomSSPin=Provided by the SPI peripheral  ActiveLowSSPin=Active low  Pin=1
      settings: SourceProductName=Embedded Coder Support Package for Texas Instruments C2000 Processors  SourceProductBaseCode=TIC2000
  Terminator : Terminator
  wires:
  value/1 -> SPI Master Transfer/1
  SPI Master Transfer/1 -> Terminator/1

== system TrailerSoftware/SPI Interface/Chart/AuxGPIO.CSHigh ==
  f : TriggerPort  TriggerType=function-call  VariantControl=(inherit)
      settings: CopyFcn=Stateflow.SLINSF.SimulinkMan.removeBlockPreDeleteFcn  PreDeleteFcn=Stateflow.SLINSF.SimulinkMan.unsafePredeleteFcn
  CS GPIO 25 : c2837xDlib/Digital Output  GPIO_Number=GPIO24~GPIO31  GPIO_Bit0=off  GPIO_BIT0_Toggle=off  GPIO_Bit1=on  GPIO_BIT1_Toggle=off  GPIO_Bit2=off  GPIO_BIT2_Toggle=off  GPIO_Bit3=off  GPIO_BIT3_Toggle=off  GPIO_Bit4=off  GPIO_BIT4_Toggle=off  GPIO_Bit5=off  GPIO_BIT5_Toggle=off  GPIO_Bit6=off  GPIO_BIT6_Toggle=off  GPIO_Bit7=off  GPIO_BIT7_Toggle=off
      settings: SourceProductName=Embedded Coder Support Package for Texas Instruments C2000 Processors  SourceProductBaseCode=TIC2000
  Constant : Constant
  wires:
  Constant/1 -> CS GPIO 25/1

== system TrailerSoftware/SPI Interface/Chart/AuxGPIO.CSLow ==
  f : TriggerPort  TriggerType=function-call  VariantControl=(inherit)
      settings: CopyFcn=Stateflow.SLINSF.SimulinkMan.removeBlockPreDeleteFcn  PreDeleteFcn=Stateflow.SLINSF.SimulinkMan.unsafePredeleteFcn
  CS GPIO 25 : c2837xDlib/Digital Output  GPIO_Number=GPIO24~GPIO31  GPIO_Bit0=off  GPIO_BIT0_Toggle=off  GPIO_Bit1=on  GPIO_BIT1_Toggle=off  GPIO_Bit2=off  GPIO_BIT2_Toggle=off  GPIO_Bit3=off  GPIO_BIT3_Toggle=off  GPIO_Bit4=off  GPIO_BIT4_Toggle=off  GPIO_Bit5=off  GPIO_BIT5_Toggle=off  GPIO_Bit6=off  GPIO_BIT6_Toggle=off  GPIO_Bit7=off  GPIO_BIT7_Toggle=off
      settings: SourceProductName=Embedded Coder Support Package for Texas Instruments C2000 Processors  SourceProductBaseCode=TIC2000
  Constant : Constant  Value=0
  wires:
  Constant/1 -> CS GPIO 25/1

== system TrailerSoftware/SPI Interface/Chart/Data ==
  value : Inport  OutDataTypeStr=uint16  PortDimensions=1
  f : TriggerPort  TriggerType=function-call  VariantControl=(inherit)
      settings: CopyFcn=Stateflow.SLINSF.SimulinkMan.removeBlockPreDeleteFcn  PreDeleteFcn=Stateflow.SLINSF.SimulinkMan.unsafePredeleteFcn
  SPI Master Transfer2 : c280xlib/SPI Master Transfer  SPISelect=SPI_A  ClockPolarity=Rising_edge  ClockPhase=No_delay  SPIModule=uint32(0)  Mode=Master  BusSpeed=uint32(1000000)  FirstBitToTransfer=Most significant bit (MSB)  ClockMode=0  BlockFunction=Transfer  EnableRegisterAddress=off  RegisterAddress=0  OutputDataType=int8  OutputDataLength=1  DataBits=8  UseCustomSSPin=Provided by the SPI peripheral  ActiveLowSSPin=Active low  Pin=1
      settings: SourceProductName=Embedded Coder Support Package for Texas Instruments C2000 Processors  SourceProductBaseCode=TIC2000
  Out1 : Outport  OutDataTypeStr=uint16  PortDimensions=1
  wires:
  SPI Master Transfer2/1 -> Out1/1
  value/1 -> SPI Master Transfer2/1

== system TrailerSoftware/SPI Interface/Chart/Master1.CheckReady1 ==
  f : TriggerPort  TriggerType=function-call  VariantControl=(inherit)
      settings: CopyFcn=Stateflow.SLINSF.SimulinkMan.removeBlockPreDeleteFcn  PreDeleteFcn=Stateflow.SLINSF.SimulinkMan.unsafePredeleteFcn
  Digital Input : c2837xDlib/Digital Input  GPIO_Number=GPIO64~GPIO71  GPIO_Bit0=off  GPIO_Bit1=off  GPIO_Bit2=off  GPIO_Bit3=on  GPIO_Bit4=off  GPIO_Bit5=off  GPIO_Bit6=off  GPIO_Bit7=off  sampleTime=-1  dataType=uint16  GPIO_Bit0_Qualification=Sync to SYSCLKOUT  GPIO_Bit1_Qualification=Sync to SYSCLKOUT  GPIO_Bit2_Qualification=Sync to SYSCLKOUT  GPIO_Bit3_Qualification=Sync to SYSCLKOUT  GPIO_Bit4_Qualification=Sync to SYSCLKOUT  GPIO_Bit5_Qualification=Sync to SYSCLKOUT  GPIO_Bit6_Qualification=Sync to SYSCLKOUT  GPIO_Bit7_Qualification=Sync to SYSCLKOUT  Qualification_Period=-1
      settings: SourceProductName=Embedded Coder Support Package for Texas Instruments C2000 Processors  SourceProductBaseCode=TIC2000
  Ready : Outport  PortDimensions=1
  wires:
  Digital Input/1 -> Ready/1

== system TrailerSoftware/SPI Interface/Chart/Output ==
  f : TriggerPort  TriggerType=function-call  VariantControl=(inherit)
      settings: CopyFcn=Stateflow.SLINSF.SimulinkMan.removeBlockPreDeleteFcn  PreDeleteFcn=Stateflow.SLINSF.SimulinkMan.unsafePredeleteFcn
  SPI Master Transfer : c280xlib/SPI Master Transfer  SPISelect=SPI_A  ClockPolarity=Rising_edge  ClockPhase=No_delay  SPIModule=uint32(0)  Mode=Master  BusSpeed=uint32(1000000)  FirstBitToTransfer=Most significant bit (MSB)  ClockMode=0  BlockFunction=Transfer  EnableRegisterAddress=off  RegisterAddress=0  OutputDataType=int8  OutputDataLength=1  DataBits=8  UseCustomSSPin=Provided by the SPI peripheral  ActiveLowSSPin=Active low  Pin=1
      settings: SourceProductName=Embedded Coder Support Package for Texas Instruments C2000 Processors  SourceProductBaseCode=TIC2000
  Write : Constant  Value=hex2dec('0')  OutDataTypeStr=uint16
  Contents : Outport  OutDataTypeStr=uint16
  wires:
  Write/1 -> SPI Master Transfer/1
  SPI Master Transfer/1 -> Contents/1

== system TrailerSoftware/SPI Interface/Chart/Read ==
  f : TriggerPort  TriggerType=function-call  VariantControl=(inherit)
      settings: CopyFcn=Stateflow.SLINSF.SimulinkMan.removeBlockPreDeleteFcn  PreDeleteFcn=Stateflow.SLINSF.SimulinkMan.unsafePredeleteFcn
  Read : Constant  Priority=1  Value=hex2dec('41')  OutDataTypeStr=uint16
  SPI Master Transfer : c280xlib/SPI Master Transfer  SPISelect=SPI_A  ClockPolarity=Rising_edge  ClockPhase=No_delay  SPIModule=uint32(0)  Mode=Master  BusSpeed=uint32(1000000)  FirstBitToTransfer=Most significant bit (MSB)  ClockMode=0  BlockFunction=Transfer  EnableRegisterAddress=off  RegisterAddress=0  OutputDataType=int8  OutputDataLength=1  DataBits=8  UseCustomSSPin=Provided by the SPI peripheral  ActiveLowSSPin=Active low  Pin=1
      settings: SourceProductName=Embedded Coder Support Package for Texas Instruments C2000 Processors  SourceProductBaseCode=TIC2000
  Terminator : Terminator
  wires:
  Read/1 -> SPI Master Transfer/1
  SPI Master Transfer/1 -> Terminator/1

== system TrailerSoftware/SPI Interface/Chart/Temps.CSHighTemp1 ==
  f : TriggerPort  TriggerType=function-call  VariantControl=(inherit)
      settings: CopyFcn=Stateflow.SLINSF.SimulinkMan.removeBlockPreDeleteFcn  PreDeleteFcn=Stateflow.SLINSF.SimulinkMan.unsafePredeleteFcn
  CS GPIO 32 : c2837xDlib/Digital Output  GPIO_Number=GPIO32~GPIO39  GPIO_Bit0=on  GPIO_BIT0_Toggle=off  GPIO_Bit1=off  GPIO_BIT1_Toggle=off  GPIO_Bit2=off  GPIO_BIT2_Toggle=off  GPIO_Bit3=off  GPIO_BIT3_Toggle=off  GPIO_Bit4=off  GPIO_BIT4_Toggle=off  GPIO_Bit5=off  GPIO_BIT5_Toggle=off  GPIO_Bit6=off  GPIO_BIT6_Toggle=off  GPIO_Bit7=off  GPIO_BIT7_Toggle=off
      settings: SourceProductName=Embedded Coder Support Package for Texas Instruments C2000 Processors  SourceProductBaseCode=TIC2000
  Constant : Constant
  wires:
  Constant/1 -> CS GPIO 32/1

== system TrailerSoftware/SPI Interface/Chart/Temps.CSLowTemp1 ==
  f : TriggerPort  TriggerType=function-call  VariantControl=(inherit)
      settings: CopyFcn=Stateflow.SLINSF.SimulinkMan.removeBlockPreDeleteFcn  PreDeleteFcn=Stateflow.SLINSF.SimulinkMan.unsafePredeleteFcn
  CS GPIO 32 : c2837xDlib/Digital Output  GPIO_Number=GPIO32~GPIO39  GPIO_Bit0=on  GPIO_BIT0_Toggle=off  GPIO_Bit1=off  GPIO_BIT1_Toggle=off  GPIO_Bit2=off  GPIO_BIT2_Toggle=off  GPIO_Bit3=off  GPIO_BIT3_Toggle=off  GPIO_Bit4=off  GPIO_BIT4_Toggle=off  GPIO_Bit5=off  GPIO_BIT5_Toggle=off  GPIO_Bit6=off  GPIO_BIT6_Toggle=off  GPIO_Bit7=off  GPIO_BIT7_Toggle=off
      settings: SourceProductName=Embedded Coder Support Package for Texas Instruments C2000 Processors  SourceProductBaseCode=TIC2000
  Constant : Constant  Value=0
  wires:
  Constant/1 -> CS GPIO 32/1

== system TrailerSoftware/SPI Interface/Chart/Temps.TempCal ==
  MSB : Inport  OutDataTypeStr=uint16  PortDimensions=1
  LSB : Inport  Port=2  OutDataTypeStr=uint16  PortDimensions=1
  f : TriggerPort  TriggerType=function-call  VariantControl=(inherit)
      settings: CopyFcn=Stateflow.SLINSF.SimulinkMan.removeBlockPreDeleteFcn  PreDeleteFcn=Stateflow.SLINSF.SimulinkMan.unsafePredeleteFcn
  Bitwise Operator : simulink/Logic and Bit Operations/Bitwise Operator  logicop=AND  UseBitMask=on  BitMask=bin2dec('00000001')  BitMaskRealWorld=Stored Integer
  Bitwise Operator1 : simulink/Logic and Bit Operations/Bitwise Operator  logicop=AND  UseBitMask=off  NumInputPorts=2  BitMask=bin2dec('11011001')  BitMaskRealWorld=Stored Integer
  Shift Arithmetic : ArithShift  BitShiftNumber=8  BitShiftDirection=Left
  Shift Arithmetic1 : ArithShift  BitShiftNumber=1  BitShiftDirection=Right
  TOut : Outport  OutDataTypeStr=uint16  PortDimensions=1
  TFault : Outport  Port=2  OutDataTypeStr=uint16  PortDimensions=1
  wires:
  LSB/1 -> Bitwise Operator1/2, Bitwise Operator/1
  Bitwise Operator/1 -> TFault/1
  MSB/1 -> Shift Arithmetic/1
  Shift Arithmetic/1 -> Bitwise Operator1/1
  Bitwise Operator1/1 -> Shift Arithmetic1/1
  Shift Arithmetic1/1 -> TOut/1

== system TrailerSoftware/SPI Interface/Chart/Write ==
  f : TriggerPort  TriggerType=function-call  VariantControl=(inherit)
      settings: CopyFcn=Stateflow.SLINSF.SimulinkMan.removeBlockPreDeleteFcn  PreDeleteFcn=Stateflow.SLINSF.SimulinkMan.unsafePredeleteFcn
  SPI Master Transfer : c280xlib/SPI Master Transfer  SPISelect=SPI_A  ClockPolarity=Rising_edge  ClockPhase=No_delay  SPIModule=uint32(0)  Mode=Master  BusSpeed=uint32(1000000)  FirstBitToTransfer=Most significant bit (MSB)  ClockMode=0  BlockFunction=Transfer  EnableRegisterAddress=off  RegisterAddress=0  OutputDataType=int8  OutputDataLength=1  DataBits=8  UseCustomSSPin=Provided by the SPI peripheral  ActiveLowSSPin=Active low  Pin=1
      settings: SourceProductName=Embedded Coder Support Package for Texas Instruments C2000 Processors  SourceProductBaseCode=TIC2000
  Terminator : Terminator
  Write : Constant  Value=hex2dec('40')  OutDataTypeStr=uint16
  wires:
  SPI Master Transfer/1 -> Terminator/1
  Write/1 -> SPI Master Transfer/1

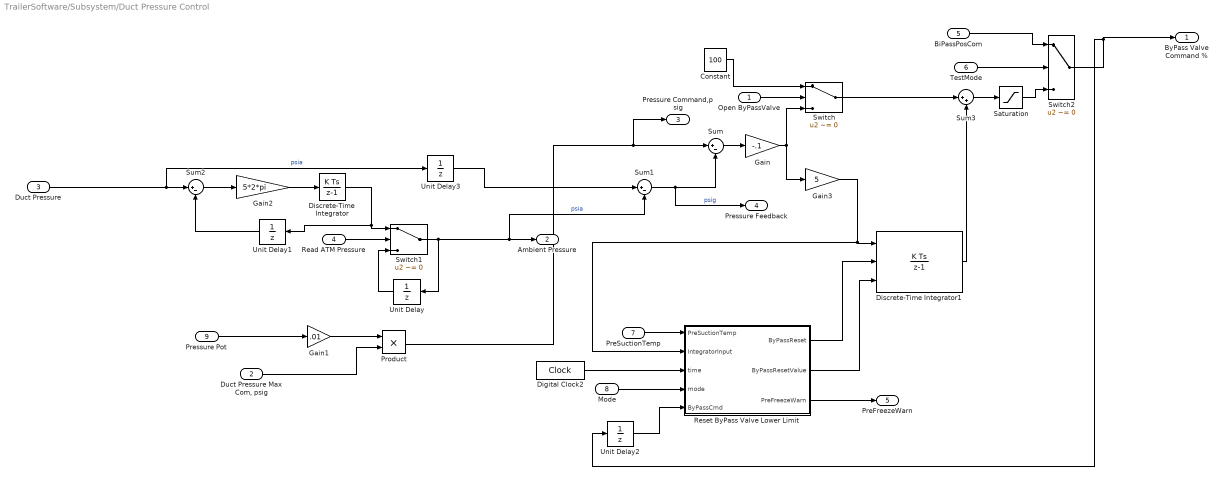
== system TrailerSoftware/Subsystem/Duct Pressure Control ==
  Open ByPassValve : Inport
  "Duct Pressure Max Com, psig" : Inport  Port=2
  Duct Pressure : Inport  Port=3
  Read ATM Pressure : Inport  Port=4
  BiPassPosCom : Inport  Port=5
  TestMode : Inport  Port=6
  PreSuctionTemp : Inport  Port=7
  Mode : Inport  Port=8
  Pressure Pot : Inport  Port=9
  Constant : Constant  Value=100
  Digital Clock2 : DigitalClock  SampleTime=update
  Discrete-Time Integrator : DiscreteIntegrator  SampleTime=-1  ICPrevOutput=DiscIntNeverNeededParam  ICPrevScaledInput=DiscIntNeverNeededParam
  Discrete-Time Integrator1 : DiscreteIntegrator  ExternalReset=level  InitialConditionSource=external  SampleTime=-1  LimitOutput=on  UpperSaturationLimit=100  LowerSaturationLimit=0  ICPrevOutput=DiscIntNeverNeededParam  ICPrevScaledInput=DiscIntNeverNeededParam
  Gain : Gain  Gain=-.1
  Gain1 : Gain  Gain=.01
  Gain2 : Gain  Gain=5*2*pi
  Gain3 : Gain  Gain=5
  Product : Product
  Reset ByPass Valve Lower Limit : MATLAB Function  TreatAsAtomicUnit=on
  Saturation : Saturate  UpperLimit=100  LowerLimit=0
  Sum : Sum  Inputs=|+-
  Sum1 : Sum  Inputs=|+-
  Sum2 : Sum  Inputs=|+-
  Sum3 : Sum  Inputs=|++
  Switch : Switch  Criteria=u2 ~= 0
  Switch1 : Switch  Criteria=u2 ~= 0
  Switch2 : Switch  Criteria=u2 ~= 0
  Unit Delay{,1..3} (4 alike) : UnitDelay  SampleTime=-1  HasFrameUpgradeWarning=on
  "ByPass Valve Command % " : Outport  VectorParamsAs1DForOutWhenUnconnected=off
  Ambient Pressure : Outport  Port=2  VectorParamsAs1DForOutWhenUnconnected=off
  Pressure Command,psig : Outport  Port=3  VectorParamsAs1DForOutWhenUnconnected=off
  Pressure Feedback : Outport  Port=4  VectorParamsAs1DForOutWhenUnconnected=off
  PreFreezeWarn : Outport  Port=5  VectorParamsAs1DForOutWhenUnconnected=off
  wires:
  Open ByPassValve/1 -> Switch/2
  Sum/1 -> Gain/1
  Duct Pressure/1 -> Unit Delay3/1, Sum2/1  "psia"
  Read ATM Pressure/1 -> Switch1/2
  Discrete-Time Integrator/1 -> Unit Delay1/1, Switch1/1
  Switch1/1 -> Sum1/2, Ambient Pressure/1, Unit Delay/1  "psia"
  Unit Delay/1 -> Switch1/3
  Pressure Pot/1 -> Gain1/1
  Gain1/1 -> Product/1
  "Duct Pressure Max Com, psig"/1 -> Product/2
  Product/1 -> Pressure Command,psig/1, Sum/1
  Sum1/1 -> Pressure Feedback/1, Sum/2  "psig"
  Unit Delay1/1 -> Sum2/2
  Gain2/1 -> Discrete-Time Integrator/1
  Sum2/1 -> Gain2/1
  BiPassPosCom/1 -> Switch2/1
  TestMode/1 -> Switch2/2
  Gain/1 -> Switch/3, Gain3/1
  Constant/1 -> Switch/1
  Switch2/1 -> "ByPass Valve Command % "/1, Unit Delay2/1
  Switch/1 -> Sum3/1
  Gain3/1 -> Reset ByPass Valve Lower Limit/2(IntegratorInput), Discrete-Time Integrator1/1
  Discrete-Time Integrator1/1 -> Sum3/2
  Sum3/1 -> Saturation/1
  Saturation/1 -> Switch2/3
  PreSuctionTemp/1 -> Reset ByPass Valve Lower Limit/1(PreSuctionTemp)
  Reset ByPass Valve Lower Limit/1(ByPassReset) -> Discrete-Time Integrator1/2
  Reset ByPass Valve Lower Limit/2(ByPassResetValue) -> Discrete-Time Integrator1/3
  Unit Delay2/1 -> Reset ByPass Valve Lower Limit/5(ByPassCmd)
  Digital Clock2/1 -> Reset ByPass Valve Lower Limit/3(time)
  Mode/1 -> Reset ByPass Valve Lower Limit/4(mode)
  Reset ByPass Valve Lower Limit/3(PreFreezeWarn) -> PreFreezeWarn/1
  Unit Delay3/1 -> Sum1/1
